simulink model "rendezvous_optimization_PSO"  (R2023a)
settings: Solver=VariableStepAuto  StartTime=0.0  StopTime=100  RelTol=1e-3
values from neighbouring files (symbols this model uses):
  Ax = [0,1;(3*(omega_T^2)),0]    [position_control.m]    (also in satellite_model.m)
  Ax_i = [0,1;0,0]    [position_control.m]    (also in satellite_model.m)
  Ay = [0,1;0,0]    [position_control.m]    (also in satellite_model.m)
  Ay_i = [0,1;0,0]    [position_control.m]    (also in satellite_model.m)
  Az = [0,1;(-(omega_T^2)),0]    [position_control.m]    (also in satellite_model.m)
  Bx = [0;1/m0]    [position_control.m]    (also in satellite_model.m)
  Bx_i = [0;1/m0]    [position_control.m]    (also in satellite_model.m)
  By = [0;1/m0]    [position_control.m]    (also in satellite_model.m)
  By_i = [0;1/m0]    [position_control.m]    (also in satellite_model.m)
  Bz = [0;1/m0]    [position_control.m]    (also in satellite_model.m)
  Cx = eye(2)    [position_control.m]    (also in satellite_model.m)
  Cx_i = eye(2)    [position_control.m]    (also in satellite_model.m)
  Cy = eye(2)    [position_control.m]    (also in satellite_model.m)
  Cy_i = eye(2)    [position_control.m]    (also in satellite_model.m)
  Cz = eye(2)    [position_control.m]    (also in satellite_model.m)
  IC_x_init = [icrf_pos_x(1);icrf_vel_x(1)]    [position_control.m]
  IC_y_init = [icrf_pos_y(2);icrf_vel_y(2)]    [position_control.m]
  m0 = 4    [position_control.m]    (also in satellite_model.m)
  mDot = 0.000102    [position_control.m]    (also in satellite_model.m)
  OC_x_init = [hill_pos_x(1);hill_vel_x(1)]    [position_control.m]
  OC_y_init = [hill_pos_y(2);hill_vel_y(2)]    [position_control.m]
  OC_z_init = [hill_pos_z(3);hill_vel_z(3)]    [position_control.m]
  omega_T = deg2rad(0.1)    [position_control.m]    (also in satellite_model.m)
  Ve = [Ve_x; 0; 0]    [position_control.m]    (also in satellite_model.m)
undefined symbols (not defined in the file or in its folder): juliandate
(part 2 of 2)

== matlab function rendezvous_optimization_PSO/Deputy Spacecraft/Guidance and Control/Control/Translational Controller/Outer Controller-x/Controller-1/MATLAB Function ==
  settings: updateMethod=DISCRETE
  data: bestKi output; bestKp output; bestKd output; error input
function [bestKi,bestKp,bestKd] = pso(error)
%% PSO_PID_Tuning.m
%----------------------------------------------------------------------
% Particle Swarm Optimization for PID Tuning


%% 2) PSO parameters
nParticles = 100;             % swarm size
Max_iter   = 100;            % iterations
dim        = 3;              % tuning [Kp, Ki, Kd]
lb         = [0   0   0];    % lower bounds
ub         = [30  20  30];    % upper bounds

w_max = 0.9; w_min = 0.4;    % inertia weight limits
c1 = 2; c2 = 2;              % cognitive and social coefficients

%% 3) Run PSO
bestGains = runPSO(error, nParticles, Max_iter, lb, ub, w_max, w_min, c1, c2);
bestKp = bestGains(1);
bestKi = bestGains(2);
bestKd = bestGains(3);


%==========================================================================
% runPSO: core Particle Swarm Optimization
%==========================================================================
function bestGains = runPSO(error, nParticles, Max_iter, lb, ub, w_max, w_min, c1, c2)
    dim = numel(lb);
    % Initialize particle positions and velocities
    pos = rand(nParticles,dim).*(ub-lb) + lb;
    vel = zeros(nParticles,dim);
    % Evaluate initial fitness
    fitness = zeros(nParticles,1);
    for i = 1:nParticles
        fitness(i) = error;
    end
    % Personal bests
    pBestPos = pos;
    pBestFit = fitness;
    % Global best
    [gBestFit, idx] = min(pBestFit);
    gBestPos = pBestPos(idx,:);

    for iter = 1:Max_iter
        % Update inertia weight linearly
        w = w_max - (w_max - w_min)*(iter/Max_iter);
        for i = 1:nParticles
            % Update velocity
            r1 = rand(1,dim);
            r2 = rand(1,dim);
            vel(i,:) = w*vel(i,:) ...
                     + c1*r1.*(pBestPos(i,:)-pos(i,:)) ...
                     + c2*r2.*(gBestPos   -pos(i,:));
            % Update position
            pos(i,:) = pos(i,:) + vel(i,:);
            % Clamp to bounds
            pos(i,:) = max(min(pos(i,:), ub), lb);
            vel(i,:) = max(min(vel(i,:), ub-lb), -(ub-lb));
            % Evaluate fitness
            fit = error;
            % Update personal best
            if fit < pBestFit(i)
                pBestFit(i) = fit;
                pBestPos(i,:) = pos(i,:);
            end
            % Update global best
            if fit < gBestFit
                gBestFit = fit;
                gBestPos = pos(i,:);
            end
        end
    end
    bestGains = gBestPos;
end

  
end

== matlab function rendezvous_optimization_PSO/Deputy Spacecraft/Guidance and Control/Control/Translational Controller/Inner Controller-z/Subsystem/MATLAB Function ==
  settings: updateMethod=DISCRETE
  data: bestKi output; bestKp output; bestKd output; error input
function [bestKi,bestKp,bestKd] = pso(error)
%% PSO_PID_Tuning.m
%----------------------------------------------------------------------
% Particle Swarm Optimization for PID Tuning


%% 2) PSO parameters
nParticles = 100;             % swarm size
Max_iter   = 100;            % iterations
dim        = 3;              % tuning [Kp, Ki, Kd]
lb         = [0   0   0];    % lower bounds
ub         = [10  5  10];    % upper bounds

w_max = 0.9; w_min = 0.4;    % inertia weight limits
c1 = 2; c2 = 2;              % cognitive and social coefficients

%% 3) Run PSO
bestGains = runPSO(error, nParticles, Max_iter, lb, ub, w_max, w_min, c1, c2);
bestKp = bestGains(1);
bestKi = bestGains(2);
bestKd = bestGains(3);


%==========================================================================
% runPSO: core Particle Swarm Optimization
%==========================================================================
function bestGains = runPSO(error, nParticles, Max_iter, lb, ub, w_max, w_min, c1, c2)
    dim = numel(lb);
    % Initialize particle positions and velocities
    pos = rand(nParticles,dim).*(ub-lb) + lb;
    vel = zeros(nParticles,dim);
    % Evaluate initial fitness
    fitness = zeros(nParticles,1);
    for i = 1:nParticles
        fitness(i) = error;
    end
    % Personal bests
    pBestPos = pos;
    pBestFit = fitness;
    % Global best
    [gBestFit, idx] = min(pBestFit);
    gBestPos = pBestPos(idx,:);

    for iter = 1:Max_iter
        % Update inertia weight linearly
        w = w_max - (w_max - w_min)*(iter/Max_iter);
        for i = 1:nParticles
            % Update velocity
            r1 = rand(1,dim);
            r2 = rand(1,dim);
            vel(i,:) = w*vel(i,:) ...
                     + c1*r1.*(pBestPos(i,:)-pos(i,:)) ...
                     + c2*r2.*(gBestPos   -pos(i,:));
            % Update position
            pos(i,:) = pos(i,:) + vel(i,:);
            % Clamp to bounds
            pos(i,:) = max(min(pos(i,:), ub), lb);
            vel(i,:) = max(min(vel(i,:), ub-lb), -(ub-lb));
            % Evaluate fitness
            fit = error;
            % Update personal best
            if fit < pBestFit(i)
                pBestFit(i) = fit;
                pBestPos(i,:) = pos(i,:);
            end
            % Update global best
            if fit < gBestFit
                gBestFit = fit;
                gBestPos = pos(i,:);
            end
        end
    end
    bestGains = gBestPos;
end

  
end

== matlab function rendezvous_optimization_PSO/Deputy Spacecraft/Guidance and Control/Control/Translational Controller/Inner Controller-x/Subsystem/MATLAB Function ==
  settings: updateMethod=DISCRETE
  data: bestKi output; bestKp output; bestKd output; error input
function [bestKi,bestKp,bestKd] = pso(error)
%% PSO_PID_Tuning.m
%----------------------------------------------------------------------
% Particle Swarm Optimization for PID Tuning


%% 2) PSO parameters
nParticles = 100;             % swarm size
Max_iter   = 100;            % iterations
dim        = 3;              % tuning [Kp, Ki, Kd]
lb         = [0   0   0];    % lower bounds
ub         = [10  5  10];    % upper bounds

w_max = 0.9; w_min = 0.4;    % inertia weight limits
c1 = 2; c2 = 2;              % cognitive and social coefficients

%% 3) Run PSO
bestGains = runPSO(error, nParticles, Max_iter, lb, ub, w_max, w_min, c1, c2);
bestKp = bestGains(1);
bestKi = bestGains(2);
bestKd = bestGains(3);


%==========================================================================
% runPSO: core Particle Swarm Optimization
%==========================================================================
function bestGains = runPSO(error, nParticles, Max_iter, lb, ub, w_max, w_min, c1, c2)
    dim = numel(lb);
    % Initialize particle positions and velocities
    pos = rand(nParticles,dim).*(ub-lb) + lb;
    vel = zeros(nParticles,dim);
    % Evaluate initial fitness
    fitness = zeros(nParticles,1);
    for i = 1:nParticles
        fitness(i) = error;
    end
    % Personal bests
    pBestPos = pos;
    pBestFit = fitness;
    % Global best
    [gBestFit, idx] = min(pBestFit);
    gBestPos = pBestPos(idx,:);

    for iter = 1:Max_iter
        % Update inertia weight linearly
        w = w_max - (w_max - w_min)*(iter/Max_iter);
        for i = 1:nParticles
            % Update velocity
            r1 = rand(1,dim);
            r2 = rand(1,dim);
            vel(i,:) = w*vel(i,:) ...
                     + c1*r1.*(pBestPos(i,:)-pos(i,:)) ...
                     + c2*r2.*(gBestPos   -pos(i,:));
            % Update position
            pos(i,:) = pos(i,:) + vel(i,:);
            % Clamp to bounds
            pos(i,:) = max(min(pos(i,:), ub), lb);
            vel(i,:) = max(min(vel(i,:), ub-lb), -(ub-lb));
            % Evaluate fitness
            fit = error;
            % Update personal best
            if fit < pBestFit(i)
                pBestFit(i) = fit;
                pBestPos(i,:) = pos(i,:);
            end
            % Update global best
            if fit < gBestFit
                gBestFit = fit;
                gBestPos = pos(i,:);
            end
        end
    end
    bestGains = gBestPos;
end

  
end

== matlab function rendezvous_optimization_PSO/Deputy Spacecraft/Guidance and Control/Control/Translational Controller/Outer Controller-x/Controller-1/MATLAB Function1 ==
  settings: updateMethod=DISCRETE
  data: reset input; error_percent output; error input
function error_percent = computeScheduledGain(reset,error)
% Compute gain based on percentage error using 1D look-up style logic
%
% Inputs:
%   r_des     : 3x1 desired position vector
%   r_current : 3x1 current position vector (from chaser)
%   r_init    : 3x1 initial position vector
%
% Output:
%   gain      : scalar scheduled gain

    persistent max_error;

    if reset || isempty(max_error)
        max_error = norm(error);  % store initial max error
    end
    
    e_now = norm(error);       % current error
    error_percent = (e_now / max_error)*100;       % normalized error: [0, 1]

   
end
